simulink model "AUV"  (R2020b)
settings: Solver=VariableStepAuto  StartTime=0.0  StopTime=60  FixedStep=1e-10  RelTol=1e-3
values from neighbouring files (symbols this model uses):
  B_eta = zeros(3,4)    [param.m]
  C_eta = m * C_eta    [param.m]
  eta_h0 = [0.2; -0.5; pi/18]    [param.m]
  F_h0 = feedfwd0 - feedback0    [param.m]
  kd = 6.56    [param.m]
  ki = 105    [param.m]
  kp = 42    [param.m]
  M_eta = diag([m m Iz])    [param.m]
  tuning = 0    [param.m]
  v_r0 = v_h0 - Vc0 * [cos(psi0); -sin(psi0); 0]    [param.m]
  Vc0 = (Vmin+Vmax)/2    (= 0.05)    [param.m]
settings Model: SimulationMode=accelerator  Creator=vicgd  LastModifiedBy=vicgd
settings SolverCC: MaxConsecutiveMinStep=100  AlgebraicLoopSolver=LineSearch
settings DebuggingCC: AlgebraicLoopMsg=none  UnderSpecifiedDimensionMsg=warning

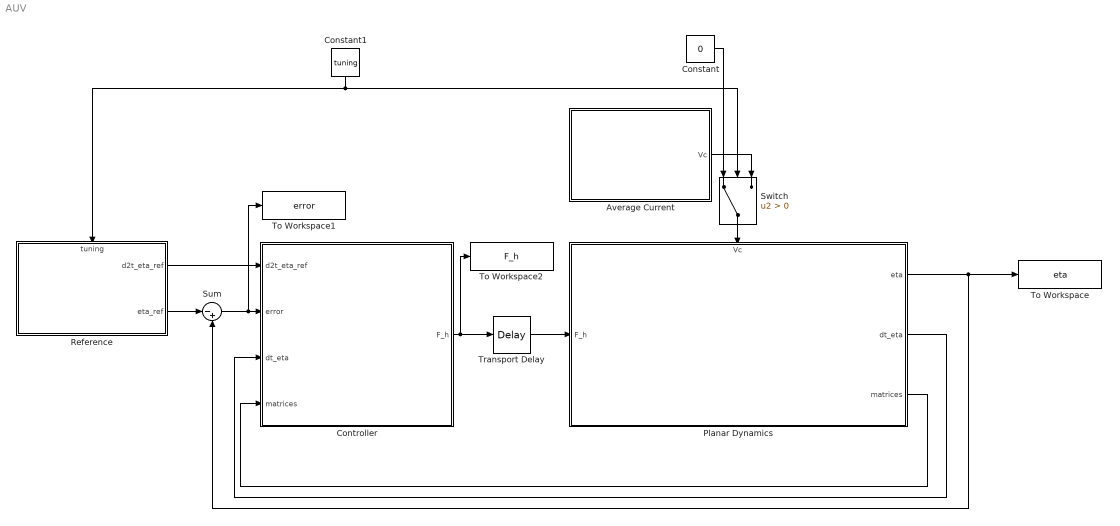
== system AUV ==
  Average Current : Subsystem
  Constant : Constant  Value=0
  Constant1 : Constant  Value=tuning
  Controller : Subsystem
      settings: MinAlgLoopOccurrences=on
  Planar Dynamics : Subsystem
      settings: MinAlgLoopOccurrences=on  PortSchema="{\"entries\":[{\"content\":{\"sides\":[{\"content\":{\"connectorIds\":[\"In1\"]},\"type\":\"ConnectorPlacement.EquallySpacedRectSide\",\"uuid\":\"0143c620-e265-4c24-b82d-29d5646815cb\"},{\"content\":{\"connectorIds\":[\"Out1\",\"Out2\",\"Out3\"],\"side\":\"RIGHT\"},\"type\":\"ConnectorPlacement.EquallySpacedRectSide\",\"uuid\":\"1c4c8258-2989-48fc-bf61-3fb3cca22766\"},{\"content\":{\"connectorIds\":[\"In2\"],\"side\":\"TOP\"},\"type\":\"ConnectorPlacement.EquallySpacedRectSide\",\"uuid\":\"b454ac2d-7a0c-4dba-924d-08c6e3fe88f8\"},{\"content\":{\"connectorIds\":[],\"side\":\"HIDDEN\"},\"type\":\"ConnectorPlacement.EquallySpacedRectSide\",\"uuid\":\"4a1c1b52-80c1-4ca2-aa18-9089299bb44a\"}]},\"type\":\"ConnectorPlacement.EquallySpacedConnector\",\"uuid\":\"9a2b1755-719e-4778-b06f-f73bd75b4848\"}],\"packageUris\":[\"http://schema.mathworks.com/mf0/Connector/R2020b\"],\"version\":\"1.0\"}"
  Reference : Subsystem
      settings: PortSchema="{\"entries\":[{\"content\":{\"sides\":[{\"content\":{\"connectorIds\":[]},\"type\":\"ConnectorPlacement.EquallySpacedRectSide\",\"uuid\":\"e30ebd2b-4078-4cb7-aeb0-aebaba51f5df\"},{\"content\":{\"connectorIds\":[\"Out1\",\"Out2\"],\"side\":\"RIGHT\"},\"type\":\"ConnectorPlacement.EquallySpacedRectSide\",\"uuid\":\"c150e25d-398d-4a19-99b1-e464475c211f\"},{\"content\":{\"connectorIds\":[\"In1\"],\"side\":\"TOP\"},\"type\":\"ConnectorPlacement.EquallySpacedRectSide\",\"uuid\":\"47b78fbd-6935-4414-8161-124ef42d7177\"},{\"content\":{\"connectorIds\":[],\"side\":\"HIDDEN\"},\"type\":\"ConnectorPlacement.EquallySpacedRectSide\",\"uuid\":\"6d2e3be9-3472-491c-90c5-a8d028e15cd2\"}]},\"type\":\"ConnectorPlacement.EquallySpacedConnector\",\"uuid\":\"029b7e70-10b3-4b56-b4d1-6d8a56368ed8\"}],\"packageUris\":[\"http://schema.mathworks.com/mf0/Connector/R2020b\"],\"version\":\"1.0\"}"
  Sum : Sum  Inputs=|-+  InputSameDT=on
  Switch : Switch  Criteria=u2 > Threshold
  To Workspace : ToWorkspace  VariableName=eta  SaveFormat=Timeseries  SampleTime=-1
  To Workspace1 : ToWorkspace  VariableName=error  SaveFormat=Timeseries  SampleTime=-1
  To Workspace2 : ToWorkspace  VariableName=F_h  SaveFormat=Timeseries  SampleTime=-1
  Transport Delay : TransportDelay  DelayTime=1e-6  InitialOutput=F_h0
  wires:
  Reference/2(eta_ref) -> Sum/1
  Reference/1(d2t_eta_ref) -> Controller/1(d2t_eta_ref)
  Sum/1 -> To Workspace1/1, Controller/2(error)
  Planar Dynamics/1(eta) -> To Workspace/1, Sum/2
  Planar Dynamics/3(matrices) -> Controller/4(matrices)
  Planar Dynamics/2(dt_eta) -> Controller/3(dt_eta)
  Average Current/1(Vc) -> Switch/3
  Switch/1 -> Planar Dynamics/2(Vc)
  Controller/1(F_h) -> Transport Delay/1, To Workspace2/1
  Transport Delay/1 -> Planar Dynamics/1(F_h)
  Constant1/1 -> Switch/2, Reference/1(tuning)
  Constant/1 -> Switch/1

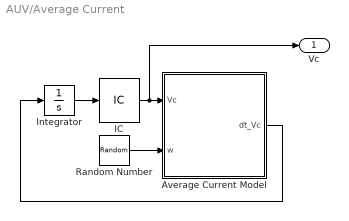
== system AUV/Average Current ==
  Average Current Model : MATLAB Function  TreatAsAtomicUnit=on
  IC : InitialCondition  Value=Vc0
  Integrator : Integrator
  Random Number : RandomNumber  SampleTime=0.1
  Vc : Outport
  wires:
  Integrator/1 -> IC/1
  Random Number/1 -> Average Current Model/2(w)
  Average Current Model/1(dt_Vc) -> Integrator/1
  IC/1 -> Vc/1, Average Current Model/1(Vc)

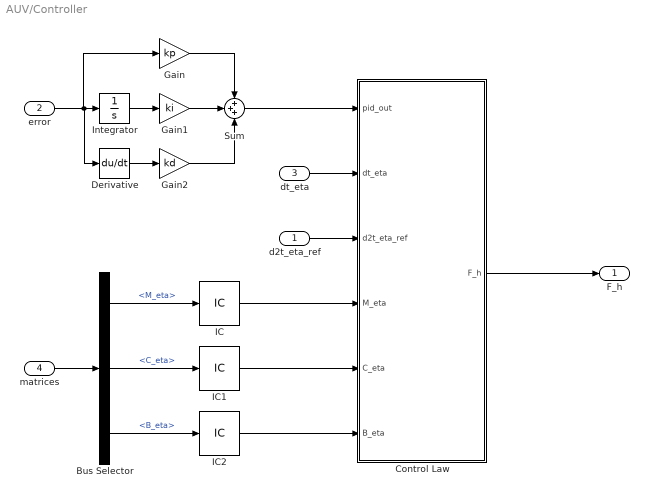
== system AUV/Controller ==
  d2t_eta_ref : Inport
  error : Inport  Port=2
  dt_eta : Inport  Port=3
  matrices : Inport  Port=4
  Bus Selector : BusSelector  OutputSignals=M_eta,C_eta,B_eta
  Control Law : MATLAB Function  TreatAsAtomicUnit=on
  Derivative : Derivative
  Gain : Gain  Gain=kp
  Gain1 : Gain  Gain=ki
  Gain2 : Gain  Gain=kd
  IC : InitialCondition  Value=M_eta
  IC1 : InitialCondition  Value=C_eta
  IC2 : InitialCondition  Value=B_eta
  Integrator : Integrator
  Sum : Sum  Inputs=+++
  F_h : Outport
  wires:
  d2t_eta_ref/1 -> Control Law/3(d2t_eta_ref)
  matrices/1 -> Bus Selector/1
  error/1 -> Gain/1, Derivative/1, Integrator/1
  Integrator/1 -> Gain1/1
  Derivative/1 -> Gain2/1
  Gain1/1 -> Sum/2
  Gain2/1 -> Sum/3
  Gain/1 -> Sum/1
  Sum/1 -> Control Law/1(pid_out)
  dt_eta/1 -> Control Law/2(dt_eta)
  Bus Selector/1 -> IC/1  "<M_eta>"
  Bus Selector/2 -> IC1/1  "<C_eta>"
  Bus Selector/3 -> IC2/1  "<B_eta>"
  IC/1 -> Control Law/4(M_eta)
  IC1/1 -> Control Law/5(C_eta)
  IC2/1 -> Control Law/6(B_eta)
  Control Law/1(F_h) -> F_h/1

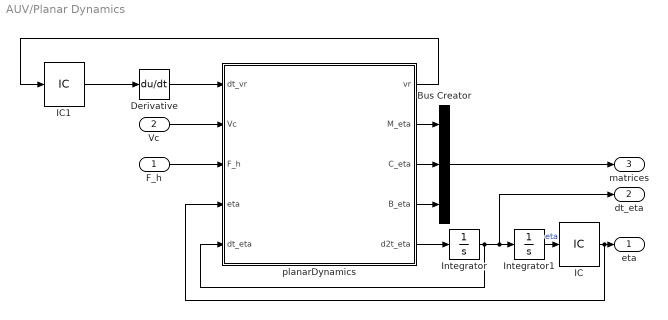
== system AUV/Planar Dynamics ==
  F_h : Inport
  Vc : Inport  Port=2
  Bus Creator : BusCreator  Inputs=3
  Derivative : Derivative
  IC : InitialCondition  Value=eta_h0
  IC1 : InitialCondition  Value=v_r0
  Integrator : Integrator
  Integrator1 : Integrator
  planarDynamics : MATLAB Function  TreatAsAtomicUnit=on
  eta : Outport
  dt_eta : Outport  Port=2
  matrices : Outport  Port=3
  wires:
  planarDynamics/5(d2t_eta) -> Integrator/1
  Vc/1 -> planarDynamics/2(Vc)
  planarDynamics/3(C_eta) -> Bus Creator/2
  Derivative/1 -> planarDynamics/1(dt_vr)
  IC1/1 -> Derivative/1
  planarDynamics/2(M_eta) -> Bus Creator/1
  planarDynamics/4(B_eta) -> Bus Creator/3
  Bus Creator/1 -> matrices/1
  Integrator/1 -> planarDynamics/5(dt_eta), dt_eta/1, Integrator1/1
  planarDynamics/1(vr) -> IC1/1
  F_h/1 -> planarDynamics/3(F_h)
  Integrator1/1 -> IC/1  "eta"
  IC/1 -> planarDynamics/4(eta), eta/1

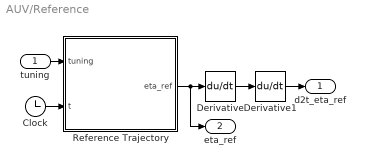
== system AUV/Reference ==
  tuning : Inport
  Clock : Clock
  Derivative : Derivative
  Derivative1 : Derivative
  Reference Trajectory : MATLAB Function  TreatAsAtomicUnit=on
  d2t_eta_ref : Outport
  eta_ref : Outport  Port=2
  wires:
  Derivative/1 -> Derivative1/1
  Reference Trajectory/1(eta_ref) -> Derivative/1, eta_ref/1
  Clock/1 -> Reference Trajectory/2(t)
  Derivative1/1 -> d2t_eta_ref/1
  tuning/1 -> Reference Trajectory/1(tuning)

== matlab function AUV/Reference/Reference Trajectory ==
  data: tuning input; t input; eta_ref output
function eta_ref = refTraj(tuning, t)
    if(tuning)
        eta_ref = [0;0;0;];
    else
        %Given 
        Rref = 1;
        rref = pi/60;
        rho0 = -pi/2;

        rho = rho0 + rref*t;
        eta_ref = [ Rref*cos(rho); 
                    Rref*(1+sin(rho));
                    pi/2 + rho];
    end

== matlab function AUV/Planar Dynamics/planarDynamics ==
  data: vr output; dt_vr input; M_eta output; C_eta output; B_eta output; Vc input; F_h input; eta input; d2t_eta output; dt_eta input
function [vr, M_eta, C_eta, B_eta, d2t_eta] = planarDynamics(dt_vr, Vc, F_h, eta, dt_eta)
    %Given 
    m = 10;
    Iz = 2;
    xg = 0.01;
    yg = 0.01;
    Lh = 0.145;
    Wh = 0.1;
    gamma = [-pi/4 pi/4 pi*3/4 -pi*3/4];
    Xu = -7.2;
    Yv = -7.7;
    Nr = -3;
    Xu_dot = -2.9;
    Yv_dot = -3;
    Nr_dot = -3.3;
    M_A = -diag([Xu_dot Yv_dot Nr_dot]);
    D_h = -diag([Xu Yv Nr]);
    
    %Unpack eta 
    psi = eta(3,1);
    
    %Helpers
    cp = cos(psi);
    sp = sin(psi);
    Jh = [ cp -sp 0;
           sp cp  0;
           0  0   1];  
    
    %Change coordinates
    vh = Jh\dt_eta;
    u = vh(1,1);
    v = vh(2,1);
    r = vh(3,1);
    
    vr = vh - Vc*[cp; -sp; 0]; %since beta = 0

    %Find M_eta
    M_eta = diag([m m Iz]);
    M_eta(1,3) = -m *(yg*cp + xg*sp);
    M_eta(2,3) = m  *(xg*cp - yg*sp);
    M_eta(3,1) = M_eta(1,3);
    M_eta(3,2) = M_eta(2,3);
    
    %Find C_eta
    C_eta = zeros(3,3);
    C_eta(1,2) = r;
    C_eta(1,3) = -cp*(v + r*xg) - sp*(u - r*yg);
    C_eta(2,1) = -r;
    C_eta(2,3) =  cp*(u - r*yg) - sp*(v + r*xg);
    C_eta(3,1) =   v*cp + u*sp;
    C_eta(3,2) = -(u*cp - v*sp);
    C_eta = m * C_eta;

    %Find B_eta
    cg = cos(gamma);
    sg = sin(gamma);
    B_eta = zeros(3,4);
    B_eta(1,1) = cos(gamma(1)+ psi);
    B_eta(2,1) = sin(gamma(1)+ psi);
    
    B_eta(1,2) = cg(2)*cp - sg(1)*sp;
    B_eta(1,3) = cg(3)*cp - sg(1)*sp;
    B_eta(1,4) = cg(4)*cp - sg(1)*sp;
    
    B_eta(2,2) = cp*sg(1) + cg(2)*sp; 
    B_eta(2,3) = cp*sg(1) + cg(3)*sp; 
    B_eta(2,4) = cp*sg(1) + cg(4)*sp; 
    
    B_eta(3,1) = -Wh*cg(1) + Lh*sg(1); 
    B_eta(3,2) =  Wh*cg(2) + Lh*sg(2); 
    B_eta(3,3) =  Wh*cg(3) - Lh*sg(3); 
    B_eta(3,4) = -Wh*cg(4) - Lh*sg(4); 
    
    %Calculate d_M
    C_hA = zeros(3,3);
    C_hA(1,3) = Yv_dot * v;
    C_hA(2,3) = -Xu_dot * u;
    C_hA(3,1) = - C_hA(1,3);
    C_hA(3,2) = - C_hA(2,3);
    
    d_M = M_eta\Jh *(-M_A*dt_vr - C_hA*vr - D_h*vr);
    
    d2t_eta = -M_eta\C_eta*dt_eta + M_eta\B_eta*F_h + d_M;

== matlab function AUV/Average Current/Average Current Model ==
  data: Vc input; dt_Vc output; w input
function dt_Vc = avgCurrent(Vc, w)
    %Given 
    Vmin = 0;
    Vmax = 0.1; 
    
    if (Vc >= Vmin) && (Vc <= Vmax)
        dt_Vc = w;
    else
        dt_Vc = -w; 
    end

== matlab function AUV/Controller/Control Law ==
  data: pid_out input; dt_eta input; d2t_eta_ref input; M_eta input; F_h output; C_eta input; B_eta input
function F_h = fcn(pid_out, dt_eta, d2t_eta_ref, M_eta, C_eta, B_eta)
    feedfwd = pinv(B_eta)*C_eta*dt_eta + pinv(B_eta)*M_eta*d2t_eta_ref;
    feedback = pinv(B_eta)*M_eta*pid_out; 
    F_h = feedfwd - feedback;
